simulink model "LevelandTemp"  (R2013a)
settings: Solver=ode45  StartTime=0.0  StopTime=10.0  RelTol=1e-3
settings Model: Creator=haresh  LastModifiedBy=haresh

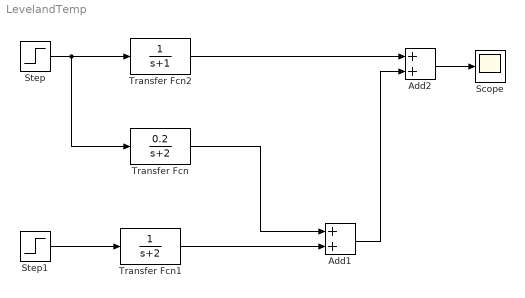
== system LevelandTemp ==
  Add1 : Sum
  Add2 : Sum
  Scope : Scope
  Step : Step  SampleTime=0
  Step1 : Step  Time=10  SampleTime=0
  Transfer Fcn : TransferFcn  Numerator=[0.2]  Denominator=[1 2]
  Transfer Fcn1 : TransferFcn  Denominator=[1 2]
  Transfer Fcn2 : TransferFcn  Denominator=[1 1]
  wires:
  Transfer Fcn/1 -> Add1/1
  Transfer Fcn1/1 -> Add1/2
  Step/1 -> Transfer Fcn/1, Transfer Fcn2/1
  Step1/1 -> Transfer Fcn1/1
  Add1/1 -> Add2/2
  Transfer Fcn2/1 -> Add2/1
  Add2/1 -> Scope/1
